simulink model "fuzzyConditioner"  (R2014a)
settings: Solver=ode45  StartTime=0.0  StopTime=100.0  RelTol=1e-3
libraries: fuzblock x2
settings Model: Creator=Aaa  LastModifiedBy=Aaa

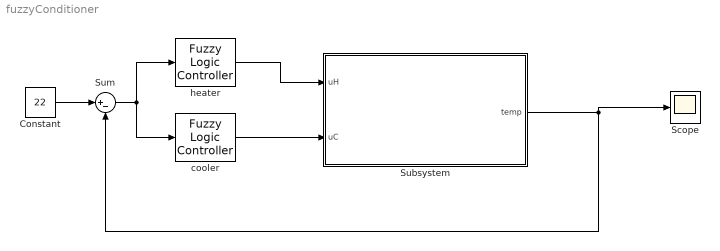
== system fuzzyConditioner ==
  Constant : Constant  Value=22
  Scope : Scope
  Subsystem : Subsystem
  Sum : Sum  Inputs=|+-
  cooler : fuzblock/Fuzzy Logic  Controller  fis='cooler'
  heater : fuzblock/Fuzzy Logic  Controller  fis='heater.fis'
  wires:
  cooler/1 -> Subsystem/2(uC)
  heater/1 -> Subsystem/1(uH)
  Subsystem/1(temp) -> Sum/2, Scope/1
  Constant/1 -> Sum/1
  Sum/1 -> cooler/1, heater/1

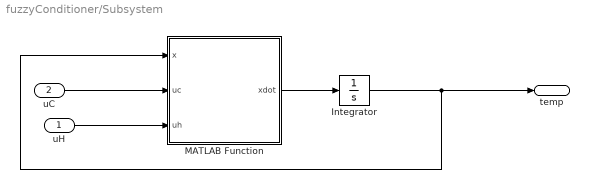
== system fuzzyConditioner/Subsystem ==
  uH : Inport
  uC : Inport  Port=2
  Integrator : Integrator
  MATLAB Function : MATLAB Function  TreatAsAtomicUnit=on
  temp : Outport
  wires:
  uC/1 -> MATLAB Function/2(uc)
  uH/1 -> MATLAB Function/3(uh)
  MATLAB Function/1(xdot) -> Integrator/1
  Integrator/1 -> MATLAB Function/1(x), temp/1

== matlab function fuzzyConditioner/Subsystem/MATLAB Function ==
  data: x input; xdot output; uc input; uh input
function xdot = fcn(x,uc,uh)
xdot=-0.1 * (x-17) - 0.5*uc + 0.5*uh;
